simulink model "Electric_vehicle_erwin"  (R2013b)
settings: Solver=ode45  StartTime=0.0  StopTime=200  MaxStep=0.001  RelTol=1e-3
undefined symbols (not defined in the file or in its folder): Ion, Lithium, sigbuilder_block
libraries: powerlib x3, electricdrivelib x1, simulink x1
settings Model: SimulationMode=accelerator  Creator=hp  LastModifiedBy=Erwin
settings DataIOCC: SignalLoggingSaveFormat=ModelDataLogs
settings OptimizationCC: BlockReduction=off  BooleanDataType=off  ExpressionDepthLimit=2147483647  InitFltsAndDblsToZero=on
settings DebuggingCC: SaveWithParameterizedLinksMsg=none  SignalResolutionControl=TryResolveAllWithWarning  SolverPrmCheckMsg=none  MultiTaskDSMMsg=warning  MultiTaskCondExecSysMsg=none  FcnCallInpInsideContextMsg=UseLocalSettings  StateNameClashWarn=warning
settings HardwareCC: TargetUnknown=on
settings SFSimCC: SimParseCustomCode=off
settings RTWCC: IncludeERTFirstTime=on
settings GRTTargetCC: TargetFcnLib=ansi_tfl_tmw.mat  CombineOutputUpdateFcns=off  GRTInterface=on
settings ConfigurationSet: Description=SimMechanics 2G

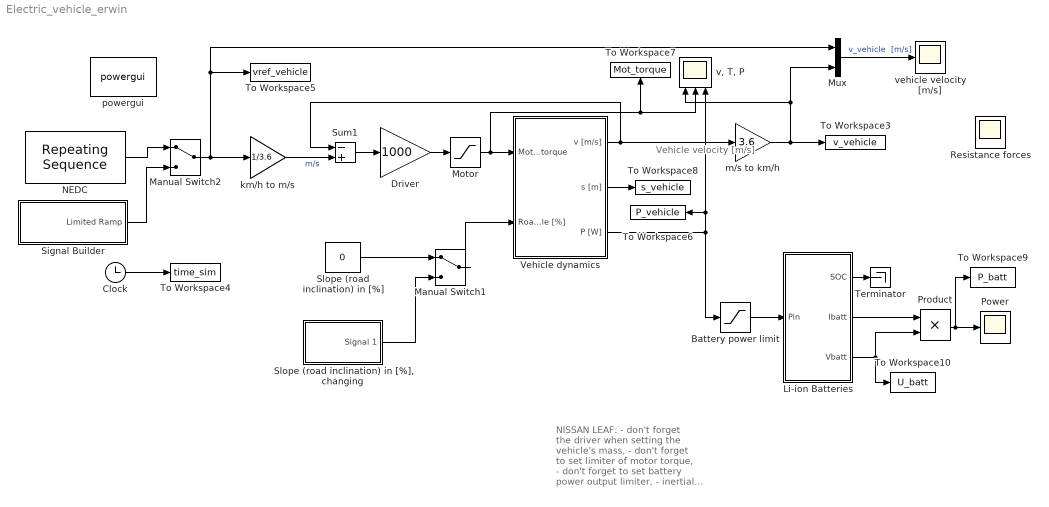
== system Electric_vehicle_erwin ==
  note: Vehicle
      | velocity [m/s]
  note: NISSAN LEAF:
      | - don't forget the driver when setting the vehicle's mass,
      | - don't forget to set limiter of motor torque,
      | - don't forget to set battery power output limiter,
      | - inertial of (all) wheels is estimated to 1.4 kg*m^2,
      | - moment of inertia of the motor shaft is estimated to 0.75 kg*m^2,
      | - use rolling resistance coefficient for concrete (0.01),
      | - don't change battery's parameters, they are pre-set.
  Battery power limit : Saturate  UpperLimit=90000  LowerLimit=0
  Clock : Clock
  Driver : Gain  Gain=1000  SaturateOnIntegerOverflow=on  OutDataTypeStr=Inherit: Same as input  ParamDataTypeStr=Inherit: Same as input
  Li-ion Batteries : Subsystem
  Manual Switch1 : ManualSwitch
  Manual Switch2 : ManualSwitch
  Motor : Saturate  UpperLimit=280  LowerLimit=0
  Mux : Mux  Inputs=2
  NEDC : simulink/Sources/Repeating Sequence  rep_seq_t=[0 12 20 25 45 60 80 90 115 135 155 165 175 182 200 212 220 225 245 260 280 290 315 335 355 365 375 382 400 412 420 425 445 460 480 490 515 535 555 565 575 582 600 612 620 625 645 660 680 690 715 735 755 765 775 782 800 825 850 910 920 990 1000 1050 1080 1120 1130 1140 1175 1200]  rep_seq_y=[0 15 15 0 0 35 35 0 0 50 50 37 37 0 0 15 15 0 0 35 35 0 0 50 50 37 37 0 0 15 15 0 0 35 35 0 0 50 50 37 37 0 0 15 15 0 0 35 35 0 0 50 50 37 37 0 0 0 70 70 50 50 70 70 100 100 120 120 0 0]
  Power : Scope
      settings: YMin=0  YMax=32.5  SaveName=ScopeData4
  Product : Product  RndMeth=Zero
  Resistance forces : Scope
      settings: YMin=0  YMax=80  SaveName=ScopeData2
  Signal Builder : Subsystem  Tag=STV Subsys  LoadFcn=sigbuilder_block('load');  StartFcn=sigbuilder_block('start');  StopFcn=sigbuilder_block('stop');  ClipboardFcn=sigbuilder_block('clipboard');  mask(Sigbuilder block){}
      mask help: Simulink:masks:SigbuilderBlock_MD
      mask init:
      | if ~strcmp(get_param(bdroot(gcbh),'SimulationStatus'),'stopped') tuvar = sigbuilder_block('maskInit'); end
      settings: CopyFcn=sigbuilder_block('copy');  DeleteFcn=sigbuilder_block('delete');  ModelCloseFcn=sigbuilder_block('modelClose');  PreSaveFcn=sigbuilder_block('preSave');  PauseFcn=sigbuilder_block('pause');  ContinueFcn=sigbuilder_block('continue');  NameChangeFcn=sigbuilder_block('namechange');  OpenFcn=sigbuilder_block('open',[437.25 199.5 591 399.75 ]);  CloseFcn=sigbuilder_block('close');
      mask Display: plot(0, 0, 100, 100,[2, 2, 32, 32, 2], [68, 8, 8, 68, 68],[32, 2], [38, 38], [32, 19, 2],[53, 60, 44], [32, 17, 17, 2],[16, 16, 31, 31]);txt = getActiveGroup(gcbh);text(2, 100, txt,'verticalAlignment', 'top');
  "Slope (road inclination) in [%], changing" : Subsystem  Tag=STV Subsys  LoadFcn=sigbuilder_block('load');  StartFcn=sigbuilder_block('start');  StopFcn=sigbuilder_block('stop');  ClipboardFcn=sigbuilder_block('clipboard');  mask(Sigbuilder block){}
      mask help: Sigbuilder GUI
      mask init:
      | if ~strcmp(get_param(bdroot(gcbh),'SimulationStatus'),'stopped') tuvar = sigbuilder_block('maskInit'); end
      settings: CopyFcn=sigbuilder_block('copy');  DeleteFcn=sigbuilder_block('delete');  ModelCloseFcn=sigbuilder_block('modelClose');  PreSaveFcn=sigbuilder_block('preSave');  PauseFcn=sigbuilder_block('pause')  ContinueFcn=sigbuilder_block('continue')  NameChangeFcn=sigbuilder_block('namechange');  OpenFcn=sigbuilder_block('open',[66 59.25 684.75 458.25 ]);  CloseFcn=sigbuilder_block('close');
      mask Display: plot(0,0,100,100,[10,10,40,40,10],[80,20,20,80,80],[40,10],[50,50], [40,27,10],[65,72,56],[40,25,25,10],[28,28,43,43]);
  Slope (road inclination) in [%] : Constant  Value=0
  Sum1 : Sum  Inputs=-+  SaturateOnIntegerOverflow=on  InputSameDT=on  OutDataTypeStr=Inherit: Same as first input
  Terminator : Terminator
  To Workspace10 : ToWorkspace  VariableName=U_batt  SampleTime=-1
  To Workspace3 : ToWorkspace  VariableName=v_vehicle  SampleTime=-1
  To Workspace4 : ToWorkspace  VariableName=time_sim  SampleTime=-1
  To Workspace5 : ToWorkspace  VariableName=vref_vehicle  SampleTime=-1
  To Workspace6 : ToWorkspace  VariableName=P_vehicle  SampleTime=-1
  To Workspace7 : ToWorkspace  VariableName=Mot_torque  SampleTime=-1
  To Workspace8 : ToWorkspace  VariableName=s_vehicle  SampleTime=-1
  To Workspace9 : ToWorkspace  VariableName=P_batt  SampleTime=-1
  Vehicle dynamics : Subsystem  mask{m_v=1601, J_motor=0.75, J_wheels=1.4, r=.2032, N=7.93, Cw=0.29, A=1.85, fr=0.01, eff_gear=0.9, v_wind=00}
      mask prompts: m_v "Vehicle mass (kg):"; J_motor "Moment of inertia of the motor's shaft [kg*m^2]:"; J_wheels "Moment of inertia of the wheels [kg*m^2]:"; r "Wheels' radius [m]:"; N "Gear ratio (transmission + final drive):"; Cw "Aerodynamic drag coefficient (kg/m):"; A "Frontal area of the vehicle [m^2]"; fr "Rolling resistance coefficient:"; eff_gear "Total efficiency of the driveline [0-1]:"; v_wind "Wind speed, negative if against the vehicle [m/s]:"
  km/h to m/s : Gain  Gain=1/3.6  SaturateOnIntegerOverflow=on  OutDataTypeStr=Inherit: Same as input  ParamDataTypeStr=Inherit: Same as input
  m/s to km/h : Gain  Gain=3.6  SaturateOnIntegerOverflow=on  OutDataTypeStr=Inherit: Same as input  ParamDataTypeStr=Inherit: Same as input
  powergui : powerlib/powergui  Priority=1  SimulationMode=Continuous  SolverType=Tustin  SampleTime=50e-6  frequency=60  SPID=off  DisableSnubberDevices=off  DisableRonSwitches=off  DisableVfSwitches=off  SwTol=0  Interpol=off  DisplayEquations=off  frequencyindice=0  Pbase=100e6  ErrMax=1e-4  Iterations=50  UnitsV=kV  UnitsW=MW  FunctionMessages=off  echomessages=off  HookPort=off  EnableUseOfTLC=off  x0status=blocks  RestoreLinks=warning  ResistiveCurrentMeasurement=off  Frange=[0:2:500]  Ylog=off  Xlog=on  ShowGrid=off  save=off  variable=ZData  ZoomFFT=off  StartTime=0.0  cycles=1  DisplayStyle=1  fundamental=60  FreqAxis=off  MaxFrequency=1000  frequencyindicesteady=1  RmsSteady=1  display=off  Ts=0  methode=off
  "v, T, P" : Scope  NumInputPorts=3
      settings: TimeRange=100  YMin=-2.5~-500~-40000  YMax=32.5~1000~150000
  vehicle velocity [m/s] : Scope
      settings: YMin=0  YMax=80
  wires:
  Mux/1 -> vehicle velocity [m/s]/1  "v_vehicle  [m/s]"
  m/s to km/h/1 -> Mux/2, "v, T, P"/1, To Workspace3/1
  Vehicle dynamics/1(v [m/s]) -> m/s to km/h/1, Sum1/1
  Vehicle dynamics/3(P [W]) -> "v, T, P"/3, To Workspace6/1, Battery power limit/1
  Sum1/1 -> Driver/1
  km/h to m/s/1 -> Sum1/2  "m/s"
  Clock/1 -> To Workspace4/1
  Vehicle dynamics/2(s [m]) -> To Workspace8/1
  Driver/1 -> Motor/1
  Manual Switch1/1 -> Vehicle dynamics/2(Road angle [%])
  Slope (road inclination) in [%]/1 -> Manual Switch1/1
  "Slope (road inclination) in [%], changing"/1(Signal 1) -> Manual Switch1/2
  Motor/1 -> Vehicle dynamics/1(Motor torque), "v, T, P"/2, To Workspace7/1
  Li-ion Batteries/3(Vbatt) -> To Workspace10/1, Product/2
  Product/1 -> Power/1, To Workspace9/1
  Li-ion Batteries/2(Ibatt) -> Product/1
  Battery power limit/1 -> Li-ion Batteries/1(Pin)
  Li-ion Batteries/1(SOC) -> Terminator/1
  Manual Switch2/1 -> To Workspace5/1, Mux/1, km/h to m/s/1
  Signal Builder/1(Limited Ramp) -> Manual Switch2/2
  NEDC/1 -> Manual Switch2/1

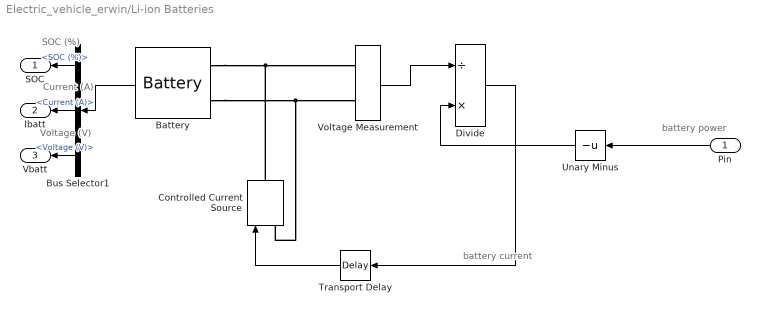
== system Electric_vehicle_erwin/Li-ion Batteries ==
  note: battery current
  note: battery power
  note: SOC (%)
  note: Current (A)
  note: Voltage (V)
  Pin : Inport
  Battery : electricdrivelib/Extra Sources/Battery  BatType=Lithium-Ion  ShowDetailedParameters=off  NomV=182  NomQ=131  SOC=100  PresetModel=on  MaxQ=131  FullV=211.8457  Dis_rate=56.9565  R=0.013893  Normal_OP=118.4696  expZone="[196.6302      6.436087]"  Dis_Char=off  current=[1.5 3]  Units=Ampere-hour  Batt_Tr=30
  Bus Selector1 : BusSelector  OutputSignals=SOC (%),Current (A),Voltage (V)
  Controlled Current Source : powerlib/Electrical Sources/Controlled Current Source  Initialize=on  Source_Type=AC  Amplitude=0  Phase=0  Frequency=0  Measurements=None
  Divide : Product  Inputs=/*
  Transport Delay : TransportDelay  DelayTime=0.01
  Unary Minus : UnaryMinus
  Voltage Measurement : powerlib/Measurements/Voltage Measurement  PhasorSimulation=off  OutputType=Complex  PSBequivalent=0
  SOC : Outport
  Ibatt : Outport  Port=2
  Vbatt : Outport  Port=3
  wires:
  Transport Delay/1 -> Controlled Current Source/1
  Voltage Measurement/1 -> Divide/1
  Divide/1 -> Transport Delay/1
  Battery/1 -> Bus Selector1/1
  Bus Selector1/1 -> SOC/1  "<SOC (%)>"
  Bus Selector1/2 -> Ibatt/1  "<Current (A)>"
  Bus Selector1/3 -> Vbatt/1  "<Voltage (V)>"
  Pin/1 -> Unary Minus/1
  Unary Minus/1 -> Divide/2
  connections:
  Battery/LConn1 -- Voltage Measurement/LConn1 -- Controlled Current Source/RConn1
  Battery/LConn2 -- Voltage Measurement/LConn2 -- Controlled Current Source/LConn1

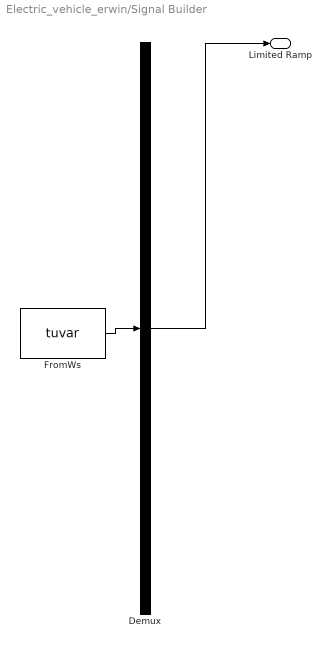
== system Electric_vehicle_erwin/Signal Builder ==
  Demux : Demux  Tag=STV Demux  Outputs=1
  FromWs : FromWorkspace  Tag=STV FromWs  VariableName=tuvar  SampleTime=0  OutputAfterFinalValue=Holding final value
      SigBuilderData=|
      | common.afterFinalStr = 'Hold final value'
      | common.sampleTime = '0'
      | dataSet.timeRange = [0 20]
      | dataSet.name = 'Group 1'
      | sbobj.Groups.Name = 'Group 1'
      | sbobj.Groups.Signals.Name = 'Limited Ramp'
      | sbobj.Groups.Signals.XData = [0 9.9 9.9 20]
      | sbobj.Groups.Signals.YData = [96.6 96.6 0 0]
      | sbobj.Groups.TimeRange = [0 20]
  Limited Ramp : Outport  Tag=STV Outport
  wires:
  Demux/1 -> Limited Ramp/1
  FromWs/1 -> Demux/1

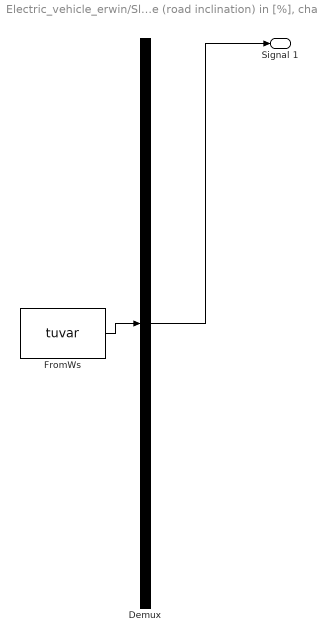
== system Electric_vehicle_erwin/Slope (road inclination) in [%], changing ==
  Demux : Demux  Tag=STV Demux  Outputs=1
  FromWs : FromWorkspace  Tag=STV FromWs  VariableName=tuvar  SampleTime=0
      SigBuilderData=|
      | common.afterFinalStr = 'Extrapolate'
      | common.sampleTime = 0
      | dataSet.timeRange = [0 100]
      | dataSet.name = 'Group 1'
      | sbobj.Groups.Name = 'Group 1'
      | sbobj.Groups.Signals.Name = 'Signal 1'
      | sbobj.Groups.Signals.XData = [0 20 40 60 80 100]
      | sbobj.Groups.Signals.YData = [0 0 1 1 0 0]
  Signal 1 : Outport  Tag=STV Outport
  wires:
  Demux/1 -> Signal 1/1
  FromWs/1 -> Demux/1

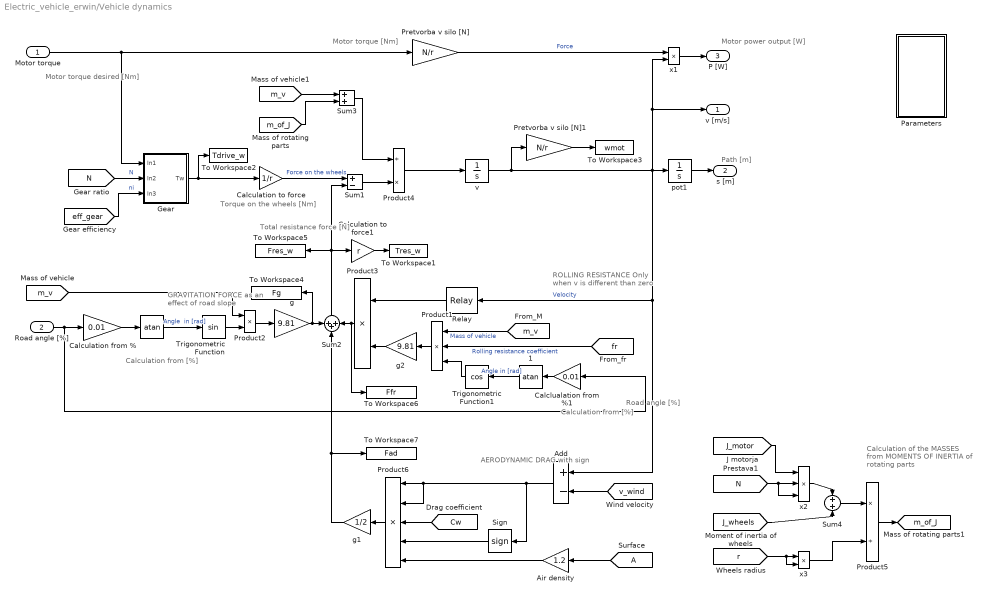
== system Electric_vehicle_erwin/Vehicle dynamics ==
  note: Path [m]
  note: ROLLING RESISTANCE
      | Only when v is different than zero
  note: AERODYNAMIC DRAG
      | with sign
  note: GRAVITATION FORCE
      | as an effect of road slope
  note: Total resistance
      | force [N]
  note: Motor
      | torque
      | desired [Nm]
  note: Torque on the
      |  wheels [Nm]
  note: Calculation of the MASSES
      | from MOMENTS OF INERTIA of
      | rotating parts
  note: Motor power output [W]
  note: Motor torque [Nm]
  note: Calculation from [%]
  note: Calculation from [%]
  note: Road angle
      | [%]
  Motor torque : Inport
  Road angle [%] : Inport  Port=2
  " " : Trigonometry  Operator=atan
  " 1" : Trigonometry  Operator=atan
  " Calculation to force" : Gain  Gain=1/r
  " Calculation to force1" : Gain  Gain=r
  Add : Sum  Inputs=+-
  Air density : Gain  Gain=1.2
  Calclualation from %1 : Gain  Gain=0.01
  Calculation from % : Gain  Gain=0.01
  Gear : Subsystem
  Parameters : Subsystem
  Pretvorba v silo [N] : Gain  Gain=N/r
  Pretvorba v silo [N]1 : Gain  Gain=N/r
  Product1 : Product  Inputs=3  SaturateOnIntegerOverflow=on  RndMeth=Zero  InputSameDT=on  OutDataTypeStr=Inherit: Same as first input
  Product2 : Product  SaturateOnIntegerOverflow=on  RndMeth=Zero  InputSameDT=on  OutDataTypeStr=Inherit: Same as first input
  Product3 : Product  SaturateOnIntegerOverflow=on  RndMeth=Zero  InputSameDT=on  OutDataTypeStr=Inherit: Same as first input
  Product4 : Product  Inputs=/*  SaturateOnIntegerOverflow=on  RndMeth=Zero  InputSameDT=on  OutDataTypeStr=Inherit: Same as first input
  Product5 : Product  Inputs=*/  SaturateOnIntegerOverflow=on  RndMeth=Zero  InputSameDT=on  OutDataTypeStr=Inherit: Same as first input
  Product6 : Product  Inputs=5  SaturateOnIntegerOverflow=on  RndMeth=Zero  InputSameDT=on  OutDataTypeStr=Inherit: Same as first input
  Relay : Relay  OnSwitchValue=.002  OffSwitchValue=.001
  Sign : Signum
  Sum1 : Sum  Inputs=+-  SaturateOnIntegerOverflow=on  InputSameDT=on  OutDataTypeStr=Inherit: Same as first input
  Sum2 : Sum  Inputs=+++  SaturateOnIntegerOverflow=on  InputSameDT=on  OutDataTypeStr=Inherit: Same as first input
  Sum3 : Sum  SaturateOnIntegerOverflow=on  InputSameDT=on  OutDataTypeStr=Inherit: Same as first input
  Sum4 : Sum  SaturateOnIntegerOverflow=on  InputSameDT=on  OutDataTypeStr=Inherit: Same as first input
  To Workspace1 : ToWorkspace  VariableName=Tres_w  SampleTime=-1
  To Workspace2 : ToWorkspace  VariableName=Tdrive_w  SampleTime=-1
  To Workspace3 : ToWorkspace  VariableName=wmot  SampleTime=-1
  To Workspace4 : ToWorkspace  VariableName=Fg  SampleTime=-1
  To Workspace5 : ToWorkspace  VariableName=Fres_w  SampleTime=-1
  To Workspace6 : ToWorkspace  VariableName=Ffr  SampleTime=-1
  To Workspace7 : ToWorkspace  VariableName=Fad  SampleTime=-1
  Trigonometric Function : Trigonometry
  Trigonometric Function1 : Trigonometry  Operator=cos
  g : Gain  Gain=9.81
  g1 : Gain  Gain=1/2
  g2 : Gain  Gain=9.81
  pot1 : Integrator
  v : Integrator
  x1 : Product  SaturateOnIntegerOverflow=on  RndMeth=Zero  InputSameDT=on  OutDataTypeStr=Inherit: Same as first input
  x2 : Product  Inputs=3  SaturateOnIntegerOverflow=on  RndMeth=Zero  InputSameDT=on  OutDataTypeStr=Inherit: Same as first input
  x3 : Product  SaturateOnIntegerOverflow=on  RndMeth=Zero  InputSameDT=on  OutDataTypeStr=Inherit: Same as first input
  v [m/s] : Outport
  s [m] : Outport  Port=2
  P [W] : Outport  Port=3
  tag scope: m_of_J=global
  wires:
  Sum2/1 -> Sum1/2, To Workspace5/1, " Calculation to force1"/1
  Trigonometric Function/1 -> Product2/2
  Product2/1 -> g/1
  pot1/1 -> s [m]/1
  v/1 -> pot1/1, x1/2, v [m/s]/1, Relay/1, Add/1, Pretvorba v silo [N]1/1  "Velocity"
  Product3/1 -> To Workspace6/1, Sum2/3
  Relay/1 -> Product3/1
  g/1 -> Sum2/1, To Workspace4/1
  [m_v] -> Product2/1
  g1/1 -> Sum2/2, To Workspace7/1
  Product6/1 -> g1/1
  [Cw] -> Product6/3
  [N] -> Gear/2(In2)  "N"
  Sum1/1 -> Product4/2
  Product4/1 -> v/1
  [m_v] -> Sum3/1
  Sum3/1 -> Product4/1
  [N] -> x2/2, x2/3
  [J_motor] -> x2/1
  [J_wheels] -> Sum4/2
  x2/1 -> Sum4/1
  Sum4/1 -> Product5/1
  Product5/1 -> [m_of_J]
  [m_of_J] -> Sum3/2
  x1/1 -> P [W]/1
  " "/1 -> Trigonometric Function/1  "Angle  in [rad]"
  Calculation from %/1 -> " "/1
  [eff_gear] -> Gear/3(In3)  "ni"
  Pretvorba v silo [N]/1 -> x1/1  "Force"
  Gear/1(Tw) -> " Calculation to force"/1, To Workspace2/1
  " Calculation to force"/1 -> Sum1/1  "Force on the wheels"
  Motor torque/1 -> Pretvorba v silo [N]/1, Gear/1(In1)
  " 1"/1 -> Trigonometric Function1/1  "Angle in [rad]"
  Calclualation from %1/1 -> " 1"/1
  Product1/1 -> g2/1
  Trigonometric Function1/1 -> Product1/3
  [fr] -> Product1/2  "Rolling resistance coefficient"
  [m_v] -> Product1/1  "Mass of vehicle"
  g2/1 -> Product3/2
  " Calculation to force1"/1 -> To Workspace1/1
  Road angle [%]/1 -> Calculation from %/1, Calclualation from %1/1
  [r] -> x3/1, x3/2
  x3/1 -> Product5/2
  Add/1 -> Product6/1, Product6/2, Sign/1
  [A] -> Air density/1
  Sign/1 -> Product6/4
  Air density/1 -> Product6/5
  [v_wind] -> Add/2
  Pretvorba v silo [N]1/1 -> To Workspace3/1

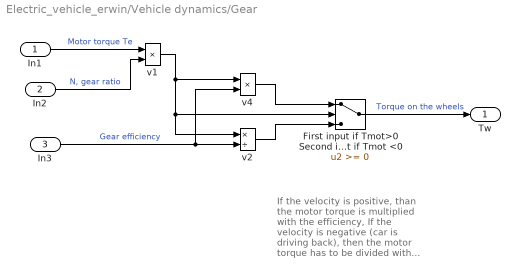
== system Electric_vehicle_erwin/Vehicle dynamics/Gear ==
  note: If the velocity is positive, than the motor torque is multiplied with the efficiency,
      | If the velocity is negative (car is driving back), then the motor torque has to be divided with the efficiency
  In1 : Inport
  In2 : Inport  Port=2
  In3 : Inport  Port=3
  First input if Tmot>0 Second input if Tmot <0 : Switch
  v1 : Product  SaturateOnIntegerOverflow=on  RndMeth=Zero  InputSameDT=on  OutDataTypeStr=Inherit: Same as first input
  v2 : Product  Inputs=*/  SaturateOnIntegerOverflow=on  RndMeth=Zero  InputSameDT=on  OutDataTypeStr=Inherit: Same as first input
  v4 : Product  SaturateOnIntegerOverflow=on  RndMeth=Zero  InputSameDT=on  OutDataTypeStr=Inherit: Same as first input
  Tw : Outport
  wires:
  In3/1 -> v2/2, v4/2  "Gear efficiency"
  v2/1 -> First input if Tmot>0 Second input if Tmot <0/3
  v4/1 -> First input if Tmot>0 Second input if Tmot <0/1
  First input if Tmot>0 Second input if Tmot <0/1 -> Tw/1  "Torque on the wheels"
  v1/1 -> v2/1, First input if Tmot>0 Second input if Tmot <0/2, v4/1
  In1/1 -> v1/1  "Motor torque Te"
  In2/1 -> v1/2  "N, gear ratio"

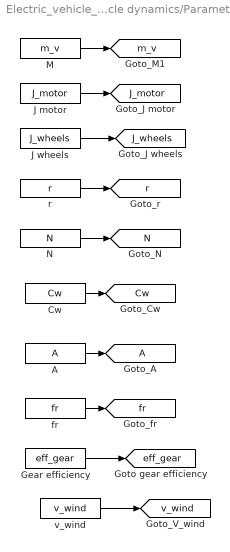
== system Electric_vehicle_erwin/Vehicle dynamics/Parameters ==
  A : Constant  Value=A
  Cw : Constant  Value=Cw
  Gear efficiency : Constant  Value=eff_gear
  J motor : Constant  Value=J_motor
  J wheels : Constant  Value=J_wheels
  M : Constant  Value=m_v
  N : Constant  Value=N
  fr : Constant  Value=fr
  r : Constant  Value=r
  v_wind : Constant  Value=v_wind
  tag scope: A=global, Cw=global, J_motor=global, J_wheels=global, N=global, eff_gear=global, fr=global, m_v=global, r=global, v_wind=global
  wires:
  N/1 -> [N]
  fr/1 -> [fr]
  Cw/1 -> [Cw]
  M/1 -> [m_v]
  J wheels/1 -> [J_wheels]
  r/1 -> [r]
  A/1 -> [A]
  J motor/1 -> [J_motor]
  Gear efficiency/1 -> [eff_gear]
  v_wind/1 -> [v_wind]
